simulink model "control"  (R2022b)
settings: Solver=VariableStepAuto  StartTime=0.0  StopTime=4  RelTol=1e-3
values from neighbouring files (symbols this model uses):
  q0 = [-0.927293431585 -1.28700579042 0.7 2.21429922201]    [generated_traj.mat]
  Tc = 0.001    [generated_traj.mat]
undefined symbols (not defined in the file or in its folder): DiscIntNeverNeededParam
settings Model: Creator=kelke  LastModifiedBy=kelke

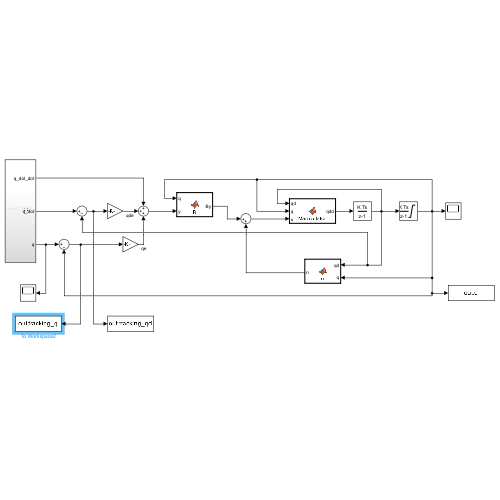
[thumbnail: Simulink's stored preview of the top-level diagram]
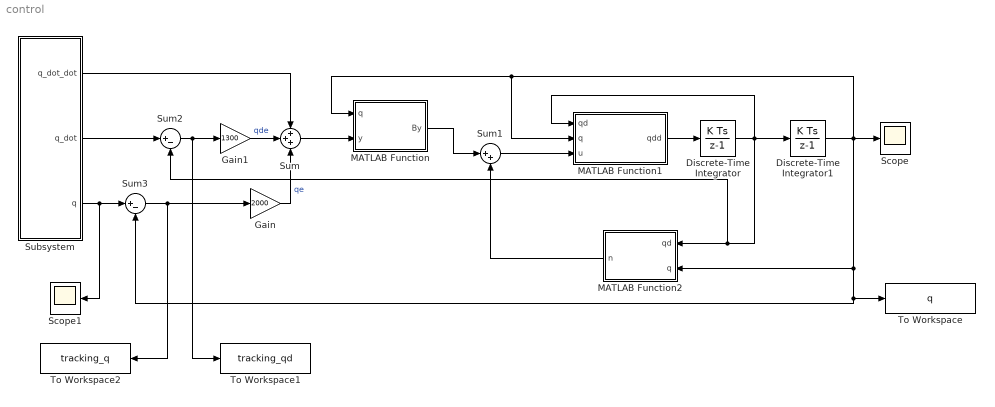
== system control ==
  Discrete-Time Integrator : DiscreteIntegrator  InitialCondition=[0;0;0;0]  SampleTime=Tc  ICPrevOutput=DiscIntNeverNeededParam  ICPrevScaledInput=DiscIntNeverNeededParam
  Discrete-Time Integrator1 : DiscreteIntegrator  InitialCondition=q0  SampleTime=Tc  LimitOutput=on  UpperSaturationLimit=[pi/2 pi/4 1 2*pi]'  LowerSaturationLimit=[-pi/2 -pi/2 0.25 -2*pi]'  ICPrevOutput=DiscIntNeverNeededParam  ICPrevScaledInput=DiscIntNeverNeededParam
  Gain : Gain  Gain=2000
  Gain1 : Gain  Gain=1300
  MATLAB Function : MATLAB Function  TreatAsAtomicUnit=on
  MATLAB Function1 : MATLAB Function  TreatAsAtomicUnit=on
  MATLAB Function2 : MATLAB Function  TreatAsAtomicUnit=on
  Scope : Scope
  Scope1 : Scope
  Subsystem : Subsystem
  Sum : Sum  Inputs=+++
  Sum1 : Sum  Inputs=|++
  Sum2 : Sum  Inputs=|+-
  Sum3 : Sum  Inputs=|+-
  To Workspace : ToWorkspace  VariableName=q  SampleTime=Tc
  To Workspace1 : ToWorkspace  VariableName=tracking_qd  SampleTime=Tc
  To Workspace2 : ToWorkspace  VariableName=tracking_q  SampleTime=Tc
  wires:
  Subsystem/1(q_dot_dot) -> Sum/1
  Subsystem/2(q_dot) -> Sum2/1
  Sum2/1 -> To Workspace1/1, Gain1/1
  Subsystem/3(q) -> Scope1/1, Sum3/1
  Sum3/1 -> To Workspace2/1, Gain/1
  Sum/1 -> MATLAB Function/2(y)
  MATLAB Function/1(By) -> Sum1/1
  MATLAB Function2/1(n) -> Sum1/2
  Sum1/1 -> MATLAB Function1/3(u)
  MATLAB Function1/1(qdd) -> Discrete-Time Integrator/1
  Discrete-Time Integrator/1 -> Discrete-Time Integrator1/1, Sum2/2, MATLAB Function2/1(qd), MATLAB Function1/1(qd)
  Discrete-Time Integrator1/1 -> Scope/1, MATLAB Function2/2(q), To Workspace/1, Sum3/2, MATLAB Function1/2(q), MATLAB Function/1(q)
  Gain/1 -> Sum/3  "qe"
  Gain1/1 -> Sum/2  "qde"

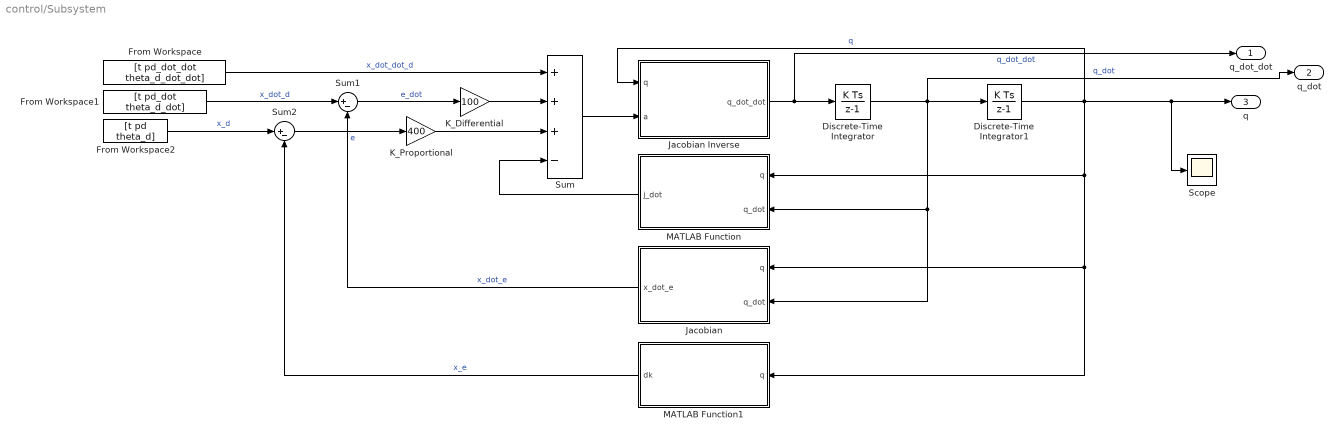
== system control/Subsystem ==
  Discrete-Time Integrator : DiscreteIntegrator  SampleTime=Tc  UpperSaturationLimit=[pi/2 pi/4 1 2*pi]'  LowerSaturationLimit=[-pi/2 -pi/2 0.25 -2*pi]'  ICPrevOutput=DiscIntNeverNeededParam  ICPrevScaledInput=DiscIntNeverNeededParam
  Discrete-Time Integrator1 : DiscreteIntegrator  InitialCondition=q0  SampleTime=Tc  LimitOutput=on  UpperSaturationLimit=[pi/2 pi/4 1 2*pi]'  LowerSaturationLimit=[-pi/2 -pi/2 0.25 -2*pi]'  ICPrevOutput=DiscIntNeverNeededParam  ICPrevScaledInput=DiscIntNeverNeededParam
  From Workspace : FromWorkspace  VariableName=[t pd_dot_dot theta_d_dot_dot]  SampleTime=Tc  OutputAfterFinalValue=Holding final value
  From Workspace1 : FromWorkspace  VariableName=[t pd_dot theta_d_dot]  SampleTime=Tc  OutputAfterFinalValue=Holding final value
  From Workspace2 : FromWorkspace  VariableName=[t pd theta_d]  SampleTime=Tc  OutputAfterFinalValue=Holding final value
  Jacobian : MATLAB Function  TreatAsAtomicUnit=on
  Jacobian Inverse : MATLAB Function  TreatAsAtomicUnit=on
  K_Differential : Gain  Gain=100
  K_Proportional : Gain  Gain=400
  MATLAB Function : MATLAB Function  TreatAsAtomicUnit=on
  MATLAB Function1 : MATLAB Function  TreatAsAtomicUnit=on
  Scope : Scope
  Sum : Sum  Inputs=+++-
  Sum1 : Sum  Inputs=|+-
  Sum2 : Sum  Inputs=|+-
  q_dot_dot : Outport
  q_dot : Outport  Port=2
  q : Outport  Port=3
  wires:
  K_Proportional/1 -> Sum/3
  Jacobian/1(x_dot_e) -> Sum1/2  "x_dot_e"
  From Workspace/1 -> Sum/1  "x_dot_dot_d"
  Discrete-Time Integrator/1 -> q_dot/1, MATLAB Function/2(q_dot), Jacobian/2(q_dot), Discrete-Time Integrator1/1  "q_dot"
  Jacobian Inverse/1(q_dot_dot) -> q_dot_dot/1, Discrete-Time Integrator/1  "q_dot_dot"
  Sum2/1 -> K_Proportional/1  "e"
  Sum1/1 -> K_Differential/1  "e_dot"
  MATLAB Function1/1(dk) -> Sum2/2  "x_e"
  K_Differential/1 -> Sum/2
  MATLAB Function/1(j_dot) -> Sum/4
  Discrete-Time Integrator1/1 -> Scope/1, q/1, MATLAB Function1/1(q), Jacobian/1(q), MATLAB Function/1(q), Jacobian Inverse/1(q)  "q"
  From Workspace2/1 -> Sum2/1  "x_d"
  Sum/1 -> Jacobian Inverse/2(a)
  From Workspace1/1 -> Sum1/1  "x_dot_d"

== matlab function control/Subsystem/Jacobian Inverse ==
  data: q input; q_dot_dot output; a input
function q_dot_dot = jacobian_inverse(q, a)

%assigning the input to joint variables
theta1 = q(1);
theta2 = q(2);
d3 = q(3);
theta4 = q(4);

%given link lengths
a1 = 0.5;
a2 = 0.5;

% homogeneous matrix from base frame to zeroth frame
HB0 = [1 0 0 0;0 1 0 0;0 0 1 1;0 0 0 1];
% homogeneous matrix from zeroth frame to first frame
H01 = [cos(theta1) -sin(theta1) 0 a1*cos(theta1);sin(theta1) cos(theta1) 0 a1*sin(theta1);0 0 1 0;0 0 0 1];
% homogeneous matrix from first frame to second frame
H12 = [cos(theta2) -sin(theta2) 0 a2*cos(theta2);sin(theta2) cos(theta2) 0 a2*sin(theta2);0 0 1 0;0 0 0 1];
% homogeneous matrix from second frame to third frame
H23 = [1 0 0 0;0 1 0 0;0 0 1 -d3;0 0 0 1];
% homogeneous matrix from third frame to fourth frame
H34 = [cos(theta4) -sin(theta4) 0 0;sin(theta4) cos(theta4) 0 0;0 0 1 0;0 0 0 1];
% homogeneous matrix from base frame to first frame
HB1 = HB0 * H01;
% homogeneous matrix from base frame to second frame
HB2 = HB1 * H12;
% homogeneous matrix from base frame to third frame
HB3 = HB2 * H23;
% homogeneous matrix from base frame to fourth frame
HB4 = (HB3 * H34);

% generating the jacobian matrix from the homogeneous matrix
z0 = [0 0 1]';
z1 = [0 0 1]';
z3 = [0 0 1]';
z2 = [0 0 1]';
p_e = HB4(1:3,4);
zP_1 = cross(z0,(p_e - [0 0 1]'));
zP_2 = cross(z1,(HB4(1:3,4) - HB1(1:3,4)));
zP_4 = cross(z3,(HB4(1:3,4) - HB3(1:3,4)));

Jacobian = [[zP_1;z0] [zP_2; z1] [z2; [0 0 0]'] [zP_4; z3]];

% making the jacobian full rank
new_Jacobian = ([Jacobian(1:3,:); Jacobian(end,:)]);
new_Jacobian(3,3)=-1;

% inverse of jacobian matrix
inv_Jacobian = (inv(new_Jacobian));

q_dot_dot = inv_Jacobian*a;

end

== matlab function control/Subsystem/Jacobian ==
  data: q input; x_dot_e output; q_dot input
function x_dot_e = jacobian(q, q_dot)

%assigning the input to joint variables
theta1 = q(1);
theta2 = q(2);
d3 = q(3);
theta4 = q(4);

%given link lengths
a1 = 0.5;
a2 = 0.5;

% homogeneous matrix from base frame to zeroth frame
HB0 = [1 0 0 0;0 1 0 0;0 0 1 1;0 0 0 1];
% homogeneous matrix from zeroth frame to first frame
H01 = [cos(theta1) -sin(theta1) 0 a1*cos(theta1);sin(theta1) cos(theta1) 0 a1*sin(theta1);0 0 1 0;0 0 0 1];
% homogeneous matrix from first frame to second frame
H12 = [cos(theta2) -sin(theta2) 0 a2*cos(theta2);sin(theta2) cos(theta2) 0 a2*sin(theta2);0 0 1 0;0 0 0 1];
% homogeneous matrix from second frame to third frame
H23 = [1 0 0 0;0 1 0 0;0 0 1 -d3;0 0 0 1];
% homogeneous matrix from third frame to fourth frame
H34 = [cos(theta4) -sin(theta4) 0 0;sin(theta4) cos(theta4) 0 0;0 0 1 0;0 0 0 1];
% homogeneous matrix from base frame to first frame
HB1 = HB0 * H01;
% homogeneous matrix from base frame to second frame
HB2 = HB1 * H12;
% homogeneous matrix from base frame to third frame
HB3 = HB2 * H23;
% homogeneous matrix from base frame to fourth frame
HB4 = (HB3 * H34);

% generating the jacobian matrix from the homogeneous matrix
z0 = [0 0 1]';
z1 = [0 0 1]';
z3 = [0 0 1]';
z2 = [0 0 1]';
p_e = HB4(1:3,4);
zP_1 = cross(z0,(p_e - [0 0 1]'));
zP_2 = cross(z1,(HB4(1:3,4) - HB1(1:3,4)));
zP_4 = cross(z3,(HB4(1:3,4) - HB3(1:3,4)));

Jacobian = [[zP_1;z0] [zP_2; z1] [z2; [0 0 0]'] [zP_4; z3]];

% making the jacobian full rank
new_Jacobian = ([Jacobian(1:3,:); Jacobian(end,:)]);
new_Jacobian(3,3)=-1;
x_dot_e = new_Jacobian*q_dot;

end

== matlab function control/Subsystem/MATLAB Function ==
  data: q input; j_dot output; q_dot input
function j_dot = jacobian_dot(q, q_dot)

% declaring variables
theta1 = q(1);
theta2 = q(2);
theta_d1 = q_dot(1);
theta_d2 = q_dot(2);

% defining the jacobian_dot function
Jacobian_dot = [- (cos(theta1)*theta_d1)/2 - (cos(theta1 + theta2)*theta_d1)/2 - (cos(theta1 + theta2)*theta_d2)/2, -(cos(theta1 + theta2)*(theta_d1 + theta_d2))/2, 0, 0; -(sin(theta1)*theta_d1)/2 - (sin(theta1 + theta2)*theta_d1)/2 - (sin(theta1 + theta2)*theta_d2)/2, -(sin(theta1 + theta2)*(theta_d1 + theta_d2))/2, 0, 0; 0,0, 0, 0; 0,0, 0, 0];

j_dot = Jacobian_dot*q_dot;
end

== matlab function control/MATLAB Function ==
  data: q input; y input; By output
function By = B(q,y)
t2=q(2);
% syms A1 A2 t1 t2 d3 t4 m1 m2 m3 m4 kr1 kr2 kr3 kr4 Il1 Il2 Il4 Im1 Im2 Im3 Im4 L1 L2 td1 td2 dd3 td4
A1 = 0.5;
A2 = 0.5;
L1 = 0.25;
L2 = 0.25;
kr1 = 1;
kr2 = 1;
kr3 = 50;
kr4 = 20;
m1 = 25;
m2 = 25;
m3 = 10;
m4 = 5;
Il1 = 5;
Il2 = 5;
Il4 = 1;
Il3 = 0;
Im1 = 0.0001;
Im2 = 0.0001;
Im3 = 0.01;
Im4 = 0.005;

%% Position
% JpM1 = [0 0 0 0; 0 0 0 0; 0 0 0 0];
% JpM2 = [-A1*sin(t1) 0 0 0; A1*cos(t1) 0 0 0; 0 0 0 0];
% JpM3 = [-A1*sin(t1)-A2*sin(t1+t2) -A2*sin(t1+t2) 0 0;A1*cos(t1)+A2*cos(t1+t2) A2*cos(t1+t2) 0 0;0 0 0 0];
% JpM4 = [-A1*sin(t1)-A2*sin(t1+t2) -A2*sin(t1+t2) 0 0;A1*cos(t1)+A2*cos(t1+t2) A2*cos(t1+t2) 0 0;0 0 0 0];
% 
% 
% JpL1 = [-L1*sin(t1) 0 0 0;L1*cos(t1) 0 0 0;0 0 0 0];
% JpL2 = [-A1*sin(t1)-L2*sin(t1+t2) -L2*sin(t1+t2) 0 0;A1*cos(t1)+L2*cos(t1+t2) L2*cos(t1+t2) 0 0;0 0 0 0];
% JpL3 = [-A1*sin(t1)-A2*sin(t1+t2) -A2*sin(t1+t2) 0 0;A1*cos(t1)+A2*cos(t1+t2) A2*cos(t1+t2) 0 0;0 0 -1 0];
% JpL4 = [-A1*sin(t1)-A2*sin(t1+t2) -A2*sin(t1+t2) 0 0;A1*cos(t1)+A2*cos(t1+t2) A2*cos(t1+t2) 0 0;0 0 1 0];
% 
%% Orientation
% 
% JoM1 = [0 0 0 0;0 0 0 0;kr1 0 0 0];
% JoM2 = [0 0 0 0;0 0 0 0;1 kr2 0 0];
% JoM3 = [0 0 0 0;0 0 0 0;1 1 -kr3 0];
% JoM4 = [0 0 0 0;0 0 0 0;1 1 0 kr4];
% 
% Jo_L1 = [0 0 0 0;0 0 0 0;1 0 0 0];
% Jo_L2 = [0 0 0 0;0 0 0 0;1 1 0 0];
% Jo_L3 = [0 0 0 0;0 0 0 0;1 1 0 0];
% Jo_L4 = [0 0 0 0;0 0 0 0; 1 1 0 1];
% 
% 
% B1 = m1*transpose(Jp_L1)*Jp_L1 + transpose(Jo_L1)*eye(3)*Il1*eye(3)'*Jo_L1 + transpose(Jo_M1)*eye(3)*Im1*eye(3)'*Jo_M1;
% B2 = m2*transpose(Jp_L2)*Jp_L2 + transpose(Jo_L2)*eye(3)*Il2*eye(3)'*Jo_L2 + transpose(Jo_M2)*eye(3)*Im2*eye(3)'*Jo_M2;
% B3 = m3*transpose(Jp_L3)*Jp_L3 + transpose(Jo_L3)*eye(3)*Il3*eye(3)'*Jo_L3 + transpose(Jo_M3)*eye(3)*Im3*eye(3)'*Jo_M3;
% B4 = m4*transpose(Jp_L4)*Jp_L4 + transpose(Jo_L4)*eye(3)*Il4*eye(3)'*Jo_L4 + transpose(Jo_M4)*eye(3)*Im4*eye(3)'*Jo_M4;
% Bn = B1+B2+B3+B4;
% B= simplify(Bn)

%% B matrix %%
B=[Il1+Il2+Il4+Im2+Im3+Im4+Im1*kr1^2+A1^2*m2+A1^2*m3+A1^2*m4+A2^2*m3+A2^2*m4+L1^2*m1+L2^2*m2+2*A1*A2*m3*cos(t2)+2*A1*A2*m4*cos(t2)+2*A1*L2*m2*cos(t2), Il2+Il4+Im3+Im4+Im2*kr2+A2^2*m3+A2^2*m4+L2^2*m2+A1*A2*m3*cos(t2)+A1*A2*m4*cos(t2)+A1*L2*m2*cos(t2), -Im3*kr3, Il4+Im4*kr4; 
   Il2+Il4+Im3+Im4+Im2*kr2+A2^2*m3+A2^2*m4+L2^2*m2+A1*A2*m3*cos(t2)+A1*A2*m4*cos(t2)+A1*L2*m2*cos(t2), Il2+Il4+Im3+Im4+Im2*kr2^2+A2^2*m3+A2^2*m4+L2^2*m2, -Im3*kr3, Il4 + Im4*kr4;
   -Im3*kr3, -Im3*kr3, Im3*kr3^2+m3+m4, 0;
   Il4+Im4*kr4, Il4+Im4*kr4, 0, Im4*kr4^2+Il4];

%% B*y matrix %%
By = B*y;

== matlab function control/MATLAB Function1 ==
  data: qd input; q input; u input; qdd output
function qdd = Manipulator(qd,q,u)
% syms A1 A2 t1 t2 d3 t4 m1 m2 m3 m4 kr1 kr2 kr3 kr4 Il1 Il2 Il4 Im1 Im2 Im3 Im4 L1 L2 td1 td2 dd3 td4
t2=q(2);
td1=qd(1);
td2=qd(2);
A1 = 0.5;
A2 = 0.5;
L1 = 0.25;
L2 = 0.25;
kr1 = 1;
kr2 = 1;
kr3 = 50;
kr4 = 20;
m1 = 25;
m2 = 25;
m3 = 10;
m4 = 5;
Il1 = 5;
Il2 = 5;
Il4 = 1;
Il3 = 0;
Im1 = 0.0001;
Im2 = 0.0001;
Im3 = 0.01;
Im4 = 0.005;
Fm1=0.0001;
Fm2=0.0001;
Fm3=0.01;
Fm4=0.005;

%% Position
% JpM1 = [0 0 0 0; 0 0 0 0; 0 0 0 0];
% JpM2 = [-A1*sin(t1) 0 0 0; A1*cos(t1) 0 0 0; 0 0 0 0];
% JpM3 = [-A1*sin(t1)-A2*sin(t1+t2) -A2*sin(t1+t2) 0 0;A1*cos(t1)+A2*cos(t1+t2) A2*cos(t1+t2) 0 0;0 0 0 0];
% JpM4 = [-A1*sin(t1)-A2*sin(t1+t2) -A2*sin(t1+t2) 0 0;A1*cos(t1)+A2*cos(t1+t2) A2*cos(t1+t2) 0 0;0 0 0 0];
% 
% 
% JpL1 = [-L1*sin(t1) 0 0 0;L1*cos(t1) 0 0 0;0 0 0 0];
% JpL2 = [-A1*sin(t1)-L2*sin(t1+t2) -L2*sin(t1+t2) 0 0;A1*cos(t1)+L2*cos(t1+t2) L2*cos(t1+t2) 0 0;0 0 0 0];
% JpL3 = [-A1*sin(t1)-A2*sin(t1+t2) -A2*sin(t1+t2) 0 0;A1*cos(t1)+A2*cos(t1+t2) A2*cos(t1+t2) 0 0;0 0 -1 0];
% JpL4 = [-A1*sin(t1)-A2*sin(t1+t2) -A2*sin(t1+t2) 0 0;A1*cos(t1)+A2*cos(t1+t2) A2*cos(t1+t2) 0 0;0 0 1 0];
% 
% %% Orientation
% 
% JoM1 = [0 0 0 0;0 0 0 0;kr1 0 0 0];
% JoM2 = [0 0 0 0;0 0 0 0;1 kr2 0 0];
% JoM3 = [0 0 0 0;0 0 0 0;1 1 -kr3 0];
% JoM4 = [0 0 0 0;0 0 0 0;1 1 0 kr4];
% 
% Jo_L1 = [0 0 0 0;0 0 0 0;1 0 0 0];
% Jo_L2 = [0 0 0 0;0 0 0 0;1 1 0 0];
% Jo_L3 = [0 0 0 0;0 0 0 0;1 1 0 0];
% Jo_L4 = [0 0 0 0;0 0 0 0; 1 1 0 1];
% 
% 
% B1 = m1*transpose(Jp_L1)*Jp_L1 + transpose(Jo_L1)*eye(3)*Il1*eye(3)'*Jo_L1 + transpose(Jo_M1)*eye(3)*Im1*eye(3)'*Jo_M1;
% B2 = m2*transpose(Jp_L2)*Jp_L2 + transpose(Jo_L2)*eye(3)*Il2*eye(3)'*Jo_L2 + transpose(Jo_M2)*eye(3)*Im2*eye(3)'*Jo_M2;
% B3 = m3*transpose(Jp_L3)*Jp_L3 + transpose(Jo_L3)*eye(3)*Il3*eye(3)'*Jo_L3 + transpose(Jo_M3)*eye(3)*Im3*eye(3)'*Jo_M3;
% B4 = m4*transpose(Jp_L4)*Jp_L4 + transpose(Jo_L4)*eye(3)*Il4*eye(3)'*Jo_L4 + transpose(Jo_M4)*eye(3)*Im4*eye(3)'*Jo_M4;
% B = B1+B2+B3+B4;
% simplify(B)

B=[Il1+Il2+Il4+Im2+Im3+Im4+Im1*kr1^2+A1^2*m2+A1^2*m3+A1^2*m4+A2^2*m3+A2^2*m4+L1^2*m1+L2^2*m2+2*A1*A2*m3*cos(t2)+2*A1*A2*m4*cos(t2)+2*A1*L2*m2*cos(t2), Il2+Il4+Im3+Im4+Im2*kr2+A2^2*m3+A2^2*m4+L2^2*m2+A1*A2*m3*cos(t2)+A1*A2*m4*cos(t2)+A1*L2*m2*cos(t2), -Im3*kr3, Il4+Im4*kr4; 
   Il2+Il4+Im3+Im4+Im2*kr2+A2^2*m3+A2^2*m4+L2^2*m2+A1*A2*m3*cos(t2)+A1*A2*m4*cos(t2)+A1*L2*m2*cos(t2), Il2+Il4+Im3+Im4+Im2*kr2^2+A2^2*m3+A2^2*m4+L2^2*m2, -Im3*kr3, Il4 + Im4*kr4;
   -Im3*kr3, -Im3*kr3, Im3*kr3^2+m3+m4, 0;
   Il4+Im4*kr4, Il4+Im4*kr4, 0, Im4*kr4^2+Il4];
% q=[t1 t2 d3 t4];
% qd=[td1 td2 dd3 td4];
% syms('C',[4 4 4]);
% syms("cf",[4 4]);
% for i=1:4
%     for j=1:4
%         for k=1:4
%             Cs(i,j,k)=0.5*diff(B(i,j),q(k))+0.5*(diff(B(i,k),q(j))-diff(B(j,k),q(i)));
%         end
%         
%     end
% end
% for x=1:4
%     for y=1:4
%         Cf(x,y)=C(x,y,1)*qd(1)+C(x,y,2)*qd(2)+C(x,y,3)*qd(3)+C(x,y,4)*qd(4);
%     end
% end 
% C=simplify(Cf)

%% C matrix %%
C=[-(55*td2*sin(t2))/8, -(55*sin(t2)*(td1 + td2))/8, 0, 0;
    (55*td1*sin(t2))/8,                           0, 0, 0;
                     0,                           0, 0, 0;
                     0,                           0, 0, 0];
%% G matrix %%
G=[0;0;-(m3+m4)*9.8;0];

%% F matrix %%
F=diag([kr1^2*Fm1 kr2^2*Fm2 kr3^3*Fm3 kr4^2*Fm4]);

%% n matrix %%
n = C*qd+F*q+G;

%% Q_dot_dot %%
qdd = inv(B)*(u-n);

== matlab function control/MATLAB Function2 ==
  data: qd input; n output; q input
function n = n(qd, q)
t2=q(2);
td1=qd(1);
td2=qd(2);
Fm1=0.0001;
Fm2=0.0001;
Fm3=0.01;
Fm4=0.005;
kr1 = 1;
kr2 = 1;
kr3 = 50;
kr4 = 20;
m1 = 25;
m2 = 25;
m3 = 10;
m4 = 5;
% q=[t1 t2 d3 t4];
% qd=[td1 td2 dd3 td4];
% syms('C',[4 4 4]);
% syms("cf",[4 4]);
% for i=1:4
%     for j=1:4
%         for k=1:4
%             Cs(i,j,k)=0.5*diff(B(i,j),q(k))+0.5*(diff(B(i,k),q(j))-diff(B(j,k),q(i)));
%         end
%         
%     end
% end
% for x=1:4
%     for y=1:4
%         Cf(x,y)=C(x,y,1)*qd(1)+C(x,y,2)*qd(2)+C(x,y,3)*qd(3)+C(x,y,4)*qd(4);
%     end
% end 
% C=simplify(Cf)

%% C Matrix %%
C=[-(55*td2*sin(t2))/8, -(55*sin(t2)*(td1 + td2))/8, 0, 0;
    (55*td1*sin(t2))/8,                           0, 0, 0;
                     0,                           0, 0, 0;
                     0,                           0, 0, 0];

%% G matrix %%
G=[0;0;-(m3+m4)*9.8;0];

%% F matrix %%
F=diag([kr1^2*Fm1 kr2^2*Fm2 kr3^3*Fm3 kr4^2*Fm4]);

%% N matrix %%
n = C*qd+F*q+G;

== matlab function control/Subsystem/MATLAB Function1 ==
  data: q input; dk output
function dk = direct_kin(q)

%assigning the input to joint variables
theta1 = q(1);
theta2 = q(2);
d3 = q(3);
theta4 = q(4);

%given link lengths
a1 = 0.5;
a2 = 0.5;

% homogeneous matrix from base frame to zeroth frame
HB0 = [1 0 0 0;0 1 0 0;0 0 1 1;0 0 0 1];
% homogeneous matrix from zeroth frame to first frame
H01 = [cos(theta1) -sin(theta1) 0 a1*cos(theta1);sin(theta1) cos(theta1) 0 a1*sin(theta1);0 0 1 0;0 0 0 1];
% homogeneous matrix from first frame to second frame
H12 = [cos(theta2) -sin(theta2) 0 a2*cos(theta2);sin(theta2) cos(theta2) 0 a2*sin(theta2);0 0 1 0;0 0 0 1];
% homogeneous matrix from second frame to third frame
H23 = [1 0 0 0;0 1 0 0;0 0 1 -d3;0 0 0 1];
% homogeneous matrix from third frame to fourth frame
H34 = [cos(theta4) -sin(theta4) 0 0;sin(theta4) cos(theta4) 0 0;0 0 1 0;0 0 0 1];
% homogeneous matrix from base frame to first frame
HB1 = HB0 * H01;
% homogeneous matrix from base frame to second frame
HB2 = HB1 * H12;
% homogeneous matrix from base frame to third frame
HB3 = HB2 * H23;
% homogeneous matrix from base frame to fourth frame
HB4 = (HB3 * H34);

% extracting position and theeta from homogeneous matrix
posx = HB4(1,4);
posy = HB4(2,4);
posz = HB4(3,4);
angleSum = theta1+theta2+theta4;


dk = [posx;posy;posz;angleSum];
end
